simulink model "PVTOL_SMC_Chattering"  (R2026b)
settings Model: Creator=nestorhernandezcastellanos  LastModifiedBy=nestorhernandezcastellanos

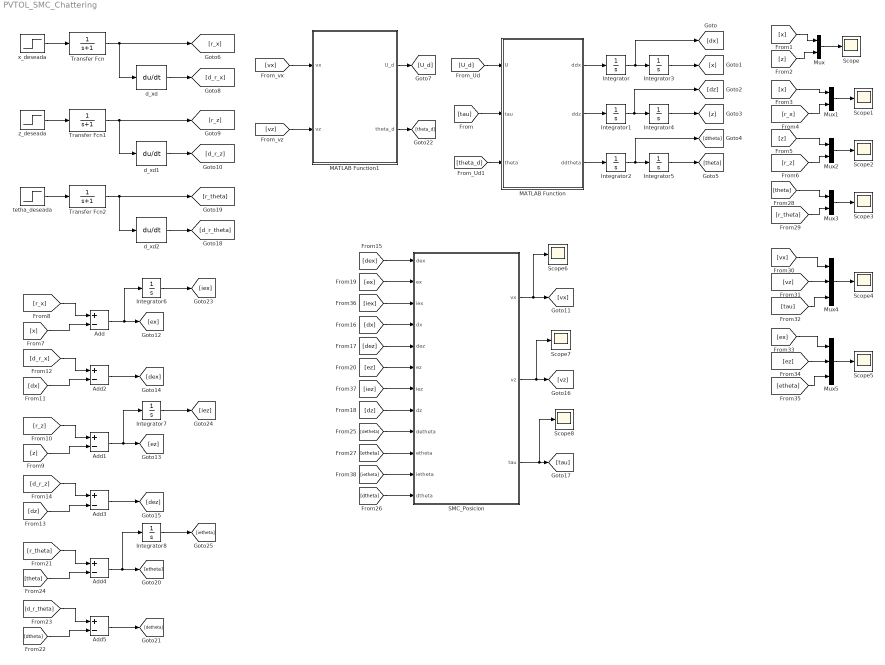
== system PVTOL_SMC_Chattering ==
  Add{,1..5} (6 alike) : Sum  Inputs=+-
  Integrator : Integrator  InitialCondition=2
  Integrator1 : Integrator  InitialCondition=3
  Integrator2 : Integrator  InitialCondition=15
  Integrator3 : Integrator  InitialCondition=2
  Integrator4 : Integrator  InitialCondition=3
  Integrator5 : Integrator  InitialCondition=15
  Integrator6 : Integrator
  Integrator7 : Integrator
  Integrator8 : Integrator
  MATLAB Function : MATLAB Function  TreatAsAtomicUnit=on
  MATLAB Function1 : MATLAB Function  TreatAsAtomicUnit=on
  Mux{,1..3} (4 alike) : Mux  Inputs=2
  Mux4 : Mux  Inputs=3
  Mux5 : Mux  Inputs=3
  SMC_Posicion : MATLAB Function  TreatAsAtomicUnit=on
  Scope{,1..8} (9 alike) : Scope
      Scope settings: ActiveDisplayYMinimum=-1.3453190171821374  ActiveDisplayYMaximum=5.7050442777254213
      Scope1 settings: ActiveDisplayYMinimum=-1.0915139503923357  ActiveDisplayYMaximum=5.6768437147487765
      Scope2 settings: ActiveDisplayYMinimum=-1.3453187915963105  ActiveDisplayYMaximum=5.7050422474529769  DataLoggingVariableName=ScopeData2
      Scope3 settings: ActiveDisplayYMinimum=-2.37928301075874  ActiveDisplayYMaximum=21.413547096828665  DataLoggingVariableName=ScopeData3
      Scope4 settings: ActiveDisplayYMinimum=-375.96530288775057  ActiveDisplayYMaximum=375.89482808407041  DataLoggingVariableName=ScopeData4
      Scope5 settings: ActiveDisplayYMinimum=-18.301916310438621  ActiveDisplayYMaximum=7.7240282277654826  DataLoggingVariableName=ScopeData5
      Scope6 settings: ActiveDisplayYMinimum=-375.96530288775057  ActiveDisplayYMaximum=375.89482808407041  DataLoggingVariableName=ScopeData6
      Scope7 settings: ActiveDisplayYMinimum=-375.96530288775057  ActiveDisplayYMaximum=375.89482808407041  DataLoggingVariableName=ScopeData7
      Scope8 settings: ActiveDisplayYMinimum=-375.96530288775057  ActiveDisplayYMaximum=375.89482808407041  DataLoggingVariableName=ScopeData8
  Transfer Fcn : TransferFcn  Denominator=[1 1]
  Transfer Fcn1 : TransferFcn  Denominator=[1 1]
  Transfer Fcn2 : TransferFcn  Denominator=[1 1]
  d_xd : Derivative
  d_xd1 : Derivative
  d_xd2 : Derivative
  tetha_deseada : Step  FinalValue=5  SampleTime=0
  x_deseada : Step  FinalValue=5  SampleTime=0
  z_deseada : Step  FinalValue=5  SampleTime=0
  wires:
  MATLAB Function/1(ddx) -> Integrator/1
  MATLAB Function/2(ddz) -> Integrator1/1
  MATLAB Function/3(ddtheta) -> Integrator2/1
  Integrator2/1 -> [dtheta], Integrator5/1
  Integrator1/1 -> [dz], Integrator4/1
  Integrator/1 -> [dx], Integrator3/1
  Integrator3/1 -> [x]
  Integrator4/1 -> [z]
  Integrator5/1 -> [theta]
  Mux/1 -> Scope/1
  [z] -> Mux/2
  [x] -> Mux/1
  x_deseada/1 -> Transfer Fcn/1
  Transfer Fcn/1 -> [r_x], d_xd/1
  [vx] -> MATLAB Function1/1(vx)
  [vz] -> MATLAB Function1/2(vz)
  [U_d] -> MATLAB Function/1(U)
  MATLAB Function1/1(U_d) -> [U_d]
  [x] -> Mux1/1
  [r_x] -> Mux1/2
  Mux1/1 -> Scope1/1
  Mux2/1 -> Scope2/1
  [r_z] -> Mux2/2
  [z] -> Mux2/1
  d_xd/1 -> [d_r_x]
  d_xd1/1 -> [d_r_z]
  Transfer Fcn1/1 -> d_xd1/1, [r_z]
  z_deseada/1 -> Transfer Fcn1/1
  [tau] -> MATLAB Function/2(tau)
  [r_x] -> Add/1
  [x] -> Add/2
  Add/1 -> Integrator6/1, [ex]
  [z] -> Add1/2
  [r_z] -> Add1/1
  Add2/1 -> [dex]
  [dx] -> Add2/2
  [d_r_x] -> Add2/1
  [d_r_z] -> Add3/1
  [dz] -> Add3/2
  Add3/1 -> [dez]
  SMC_Posicion/1(vx) -> Scope6/1, [vx]
  SMC_Posicion/2(vz) -> Scope7/1, [vz]
  SMC_Posicion/3(tau) -> Scope8/1, [tau]
  [dex] -> SMC_Posicion/1(dex)
  [dx] -> SMC_Posicion/4(dx)
  [dez] -> SMC_Posicion/5(dez)
  [dz] -> SMC_Posicion/8(dz)
  [ex] -> SMC_Posicion/2(ex)
  [ez] -> SMC_Posicion/6(ez)
  tetha_deseada/1 -> Transfer Fcn2/1
  Transfer Fcn2/1 -> [r_theta], d_xd2/1
  d_xd2/1 -> [d_r_theta]
  Add5/1 -> [detheta]
  [dtheta] -> Add5/2
  [d_r_theta] -> Add5/1
  [r_theta] -> Add4/1
  [theta] -> Add4/2
  [detheta] -> SMC_Posicion/9(detheta)
  [etheta] -> SMC_Posicion/10(etheta)
  [dtheta] -> SMC_Posicion/12(dtheta)
  MATLAB Function1/2(theta_d) -> [theta_d]
  [theta_d] -> MATLAB Function/3(theta)
  [theta] -> Mux3/1
  [r_theta] -> Mux3/2
  Mux3/1 -> Scope3/1
  Mux4/1 -> Scope4/1
  [vz] -> Mux4/2
  [vx] -> Mux4/1
  [tau] -> Mux4/3
  [etheta] -> Mux5/3
  [ex] -> Mux5/1
  [ez] -> Mux5/2
  Mux5/1 -> Scope5/1
  [iex] -> SMC_Posicion/3(iex)
  [iez] -> SMC_Posicion/7(iez)
  [ietheta] -> SMC_Posicion/11(ietheta)
  Integrator6/1 -> [iex]
  Integrator7/1 -> [iez]
  Add1/1 -> Integrator7/1, [ez]
  Add4/1 -> Integrator8/1, [etheta]
  Integrator8/1 -> [ietheta]

== matlab function PVTOL_SMC_Chattering/MATLAB Function1 ==
  data: vx input; U_d output; vz input; theta_d output
function [U_d,theta_d] = linealizacion(vx,vz)

g = 9.81;                                  
U_d = sqrt(vx^2 + (vz+g)^2);                 
theta_d = atan2(-vx,vz+g);

== matlab function PVTOL_SMC_Chattering/MATLAB Function ==
  data: U input; ddx output; tau input; theta input; ddz output; ddtheta output
function [ddx,ddz,ddtheta] = planta(U,tau,theta)

g = 9.81;                                       

ddx = -U*sin(theta);                            
ddz = U*cos(theta)-g;                           
ddtheta = tau;

== matlab function PVTOL_SMC_Chattering/SMC_Posicion ==
  data: dex input; ex input; iex input; dx input; vx output; dez input; ez input; iez input; dz input; vz output; tau output; detheta input; etheta input; ietheta input; dtheta input
function [vx, vz, tau] = controlador(dex, ex, iex, dx, dez, ez, iez, dz, detheta, etheta, ietheta, dtheta)

% Ganancias del controlador
Kx = 3;
Kz = 3;
Ktheta = 3;

% Parámetros de las superficies de deslizamiento
mx1 = 2.0;
mx2 = 2.2;

mz1 = 2.0;
mz2 = 2.2;

mtheta1 = 2.0;
mtheta2 = 2.2;

% Cotas superiores
Lx = 0.8;
Lz = 0.8;
Ltheta = 0.8;

% Superficies de deslizamiento integrales
sigma_x = dex + mx1*ex + mx2*iex;
sigma_z = dez + mz1*ez + mz2*iez;
sigma_theta = detheta + mtheta1*etheta + mtheta2*ietheta;

% Valores equivalentes
Veq_x = Lx + mx1*abs(dx) + mx2*abs(ex);
Veq_z = Lz + mz1*abs(dz) + mz2*abs(ez);
Veq_theta = Ltheta + mtheta1*abs(dtheta) + mtheta2*abs(etheta);

% Leyes de control
vx = Kx*Veq_x*sign(sigma_x);
vz = Kz*Veq_z*sign(sigma_z);
tau = Ktheta*Veq_theta*sign(sigma_theta);
